simulink model "CoffeeReactor_ex_4_2"  (R2023b)
settings: Solver=ode4  StartTime=0.0  StopTime=simulationParameters.Tsim  FixedStep=simulationParameters.Tint  RelTol=1e-3
undefined symbols (not defined in the file): futureRefCalc, I, PH, simulationParameters, sys_d, Ts
settings Model: Creator=simone  LastModifiedBy=fabiomosele
settings SolverCC: AlgebraicLoopSolver=TrustRegion
settings DataIOCC: SaveOutput=off  SignalLogging=off  DSMLogging=off  SaveTime=off  ReturnWorkspaceOutputs=off
settings DebuggingCC: UnconnectedInputMsg=warning  UnconnectedOutputMsg=warning  UnconnectedLineMsg=warning
settings ModelReferenceCC: EnableRefExpFcnMdlSchedulingChecks=on
settings RTWCC: DLArmComputeVersion=19.05

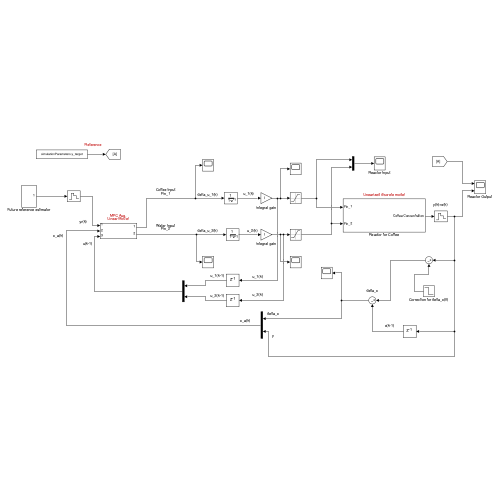
[thumbnail: Simulink's stored preview of the top-level diagram]
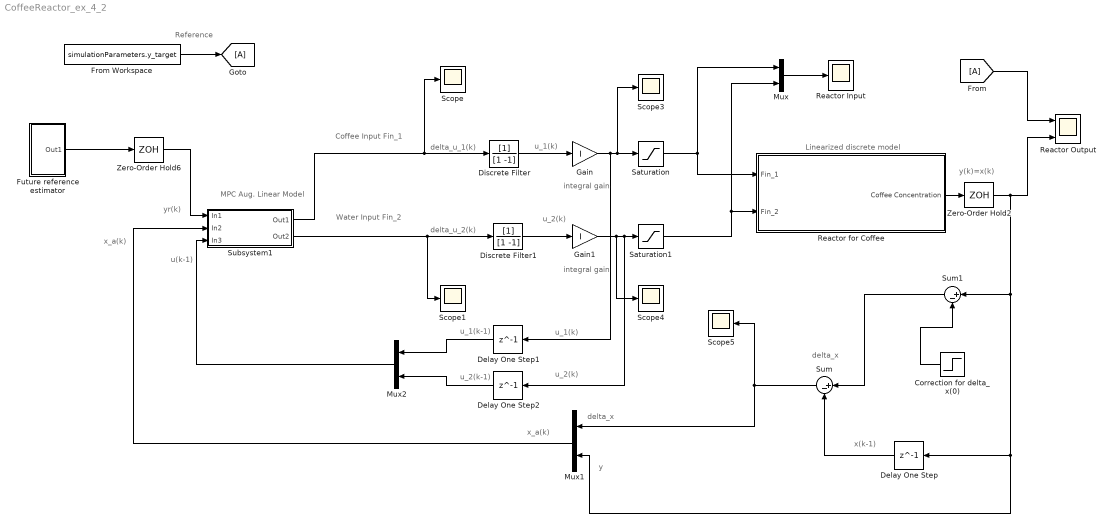
== system CoffeeReactor_ex_4_2 ==
  note: u(k-1)
  note: u_1(k)
  note: x(k-1)
  note: integral gain
  note: y
  note: delta_x
  note: delta_x
  note: u_1(k)
  note: delta_u_1(k)
  note: yr(k)
  note: Linearized discrete model
  note: Coffee Input Fin_1
  note: x_a(k)
  note: MPC Aug. Linear Model
  note: Reference
  note: y(k)=x(k)
  note: Water Input Fin_2
  note: delta_u_2(k)
  note: u_2(k)
  note: x_a(k)
  note: integral gain
  note: u_2(k)
  note: u_2(k-1)
  note: u_1(k-1)
  Correction for delta_x(0) : Step  Time=Ts  Before=simulationParameters.Reactor_parameters.x_0  After=0  SampleTime=Ts
  Delay One Step : Delay  DelayLength=1
  Delay One Step1 : Delay  DelayLength=1
  Delay One Step2 : Delay  DelayLength=1
  Discrete Filter : DiscreteFilter  Denominator=[1 -1]
  Discrete Filter1 : DiscreteFilter  Denominator=[1 -1]
  From : From
  From Workspace : FromWorkspace  VariableName=simulationParameters.y_target  OutputAfterFinalValue=Holding final value
  Future reference estimator : Subsystem
  Gain : Gain  Gain=I
  Gain1 : Gain  Gain=I
  Goto : Goto
  Mux : Mux  Inputs=2
  Mux1 : Mux  Inputs=2
  Mux2 : Mux  Inputs=2
  Reactor Input : Scope
  Reactor Output : Scope  NumInputPorts=2
  Reactor for Coffee : Subsystem
  Saturation : Saturate  UpperLimit=simulationParameters.Fin1_max  LowerLimit=simulationParameters.Fin1_min
  Saturation1 : Saturate  UpperLimit=simulationParameters.Fin2_max  LowerLimit=simulationParameters.Fin2_min
  Scope{,1,3..5} (5 alike) : Scope
  Subsystem1 : Subsystem
  Sum : Sum  Inputs=|+-
  Sum1 : Sum  Inputs=|+-
  Zero-Order Hold2 : ZeroOrderHold  SampleTime=simulationParameters.Ts
  Zero-Order Hold6 : ZeroOrderHold  SampleTime=simulationParameters.Ts
  wires:
  From/1 -> Reactor Output/1
  Mux/1 -> Reactor Input/1
  Saturation/1 -> Reactor for Coffee/1(Fin_1), Mux/1
  Saturation1/1 -> Reactor for Coffee/2(Fin_2), Mux/2
  From Workspace/1 -> Goto/1
  Delay One Step/1 -> Sum/2
  Sum/1 -> Scope5/1, Mux1/1
  Zero-Order Hold2/1 -> Delay One Step/1, Mux1/2, Sum1/1, Reactor Output/2
  Mux1/1 -> Subsystem1/2(In2)
  Subsystem1/2(Out2) -> Discrete Filter1/1, Scope1/1
  Subsystem1/1(Out1) -> Discrete Filter/1, Scope/1
  Zero-Order Hold6/1 -> Subsystem1/1(In1)
  Reactor for Coffee/1(Coffee Concentration) -> Zero-Order Hold2/1
  Correction for delta_x(0)/1 -> Sum1/2
  Sum1/1 -> Sum/1
  Discrete Filter/1 -> Gain/1
  Gain1/1 -> Delay One Step2/1, Saturation1/1, Scope4/1
  Discrete Filter1/1 -> Gain1/1
  Gain/1 -> Delay One Step1/1, Scope3/1, Saturation/1
  Future reference estimator/1(Out1) -> Zero-Order Hold6/1
  Delay One Step1/1 -> Mux2/1
  Delay One Step2/1 -> Mux2/2
  Mux2/1 -> Subsystem1/3(In3)

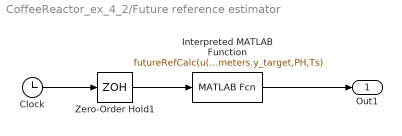
== system CoffeeReactor_ex_4_2/Future reference estimator ==
  Clock : Clock
  Interpreted MATLAB Function : MATLABFcn  MATLABFcn=futureRefCalc(u(1),simulationParameters.y_target,PH,Ts)  OutputDimensions=PH
  Zero-Order Hold1 : ZeroOrderHold  SampleTime=Ts
  Out1 : Outport
  wires:
  Interpreted MATLAB Function/1 -> Out1/1
  Clock/1 -> Zero-Order Hold1/1
  Zero-Order Hold1/1 -> Interpreted MATLAB Function/1

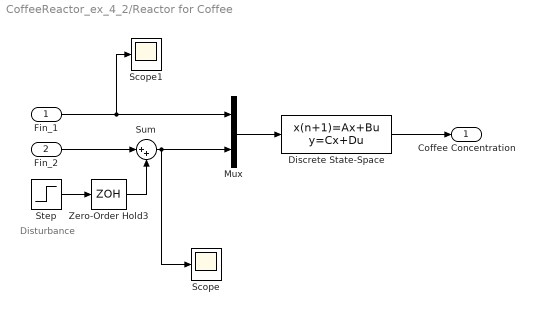
== system CoffeeReactor_ex_4_2/Reactor for Coffee ==
  note: Disturbance
  Fin_1 : Inport
  Fin_2 : Inport  Port=2
  Discrete State-Space : DiscreteStateSpace  A=sys_d.A  B=sys_d.B  C=sys_d.C  D=sys_d.D  InitialCondition=simulationParameters.Reactor_parameters.x_0  SampleTime=-1
  Mux : Mux  Inputs=2
  Scope : Scope
  Scope1 : Scope
  Step : Step  Time=simulationParameters.Reactor_parameters.Tdist  After=simulationParameters.Reactor_parameters.Adist  SampleTime=0
  Sum : Sum  Inputs=|++
  Zero-Order Hold3 : ZeroOrderHold  SampleTime=simulationParameters.Ts
  Coffee Concentration : Outport
  wires:
  Fin_1/1 -> Scope1/1, Mux/1
  Mux/1 -> Discrete State-Space/1
  Fin_2/1 -> Sum/1
  Sum/1 -> Scope/1, Mux/2
  Step/1 -> Zero-Order Hold3/1
  Zero-Order Hold3/1 -> Sum/2
  Discrete State-Space/1 -> Coffee Concentration/1

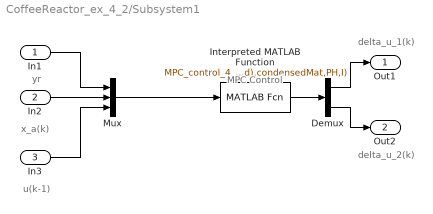
== system CoffeeReactor_ex_4_2/Subsystem1 ==
  note: u(k-1)
  note: yr
  note: x_a(k)
  note: delta_u_1(k)
  note: MPC Control
  note: delta_u_2(k)
  In1 : Inport
  In2 : Inport  Port=2
  In3 : Inport  Port=3
  Demux : Demux  Outputs=2
  Interpreted MATLAB Function : MATLABFcn  MATLABFcn=MPC_control_4_2(u(1:PH),u(PH+1:PH+2),u(PH+3:end),condensedMat,PH,I)  OutputDimensions=2
  Mux : Mux  Inputs=3
  Out1 : Outport
  Out2 : Outport  Port=2
  wires:
  Interpreted MATLAB Function/1 -> Demux/1
  Demux/2 -> Out2/1
  Demux/1 -> Out1/1
  In2/1 -> Mux/2
  In1/1 -> Mux/1
  Mux/1 -> Interpreted MATLAB Function/1
  In3/1 -> Mux/3
